simulink model "testLight"  (R2013a)
settings: Solver=ode3  SolverMode=SingleTasking  StartTime=0.0  StopTime=10.0  RelTol=1e-3
libraries: simulink x1
settings Model: ExtModeTrigDuration=2  Creator=grouleau  LastModifiedBy=grouleau
settings OptimizationCC: ExpressionDepthLimit=2147483647  OptimizeModelRefInitCode=on  LifeSpan=1
settings DebuggingCC: SolverPrmCheckMsg=none  StrictBusMsg=Warning
settings HardwareCC: ProdLargestAtomicInteger=Long  ProdLargestAtomicFloat=Float  ProdEndianess=LittleEndian  ProdHWDeviceType=ARM Compatible->ARM 7
settings RTWCC: SystemTargetFile=realtime.tlc  GenerateMakefile=off  TemplateMakefile=realtime.tmf  Description=Real-Time Toolbox  RTWVerbose=off  ProcessScript=realtime_make_rtw_hook
settings CodeAppCC: CustomSymbolStrType=$N$R$M  InternalIdentifier=Classic
settings STFCustomTargetCC: TargetLibSuffix=.a  GenerateSampleERTMain=on  ERTCustomFileBanners=on  SupportNonInlinedSFcns=off  SupportVariableSizeSignals=on  MATLABClassNameForMDSCustomization=Simulink.SoftwareTarget.ERTCustomization  SystemTargetFile=realtime.tlc
settings ERTTargetCC: ParMdlRefBuildCompliant=off  CompOptLevelCompliant=off  ConcurrentExecutionCompliant=off  CombineOutputUpdateFcns=off  ERTFirstTimeCompliant=off  SupportContinuousTime=on  SupportVariableSizeSignals=on  ModelStepFunctionPrototypeControlCompliant=off  CPPClassGenCompliant=off  ERTSrcFileBannerTemplate=realtime_code_template.cgt  ERTHdrFileBannerTemplate=realtime_code_template.cgt  ERTDataSrcFileTemplate=realtime_code_template.cgt  ERTDataHdrFileTemplate=realtime_code_template.cgt  ERTCustomFileTemplate=realtime_file_process.tlc

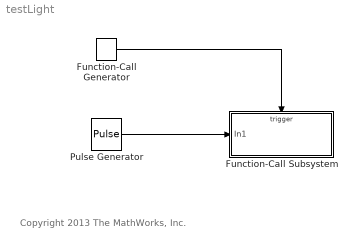
== system testLight ==
  note: Copyright 2013 The MathWorks, Inc.
  Function-Call Generator : simulink/Ports & Subsystems/Function-Call Generator  sample_time=1  numberOfIterations=1
  Function-Call Subsystem : Subsystem  TreatAsAtomicUnit=on
  Pulse Generator : DiscretePulseGenerator
  wires:
  Function-Call Generator/1 -> Function-Call Subsystem/Trigger
  Pulse Generator/1 -> Function-Call Subsystem/1(In1)

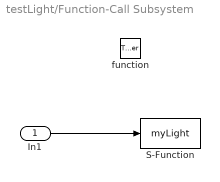
== system testLight/Function-Call Subsystem ==
  In1 : Inport
  function : TriggerPort  TriggerType=function-call
  S-Function : S-Function  FunctionName=myLight  EnableBusSupport=off
  wires:
  In1/1 -> S-Function/1
